simulink model "peak_current_mode_3phase_4quadrant"  (R2021b)
settings: Solver=VariableStepAuto  StartTime=0.0  StopTime=100  RelTol=1e-3
libraries: spsUniversalBridgeLib x2, spsCurrentMeasurementLib x1, spsDCMachineLib x1, spsDCVoltageSourceLib x1, spsThreePhaseVIMeasurementLib x1, spsThreePhaseSourceLib x1, spspowerguiLib x1
settings Model: Creator=Göktuğ  LastModifiedBy=Göktuğ

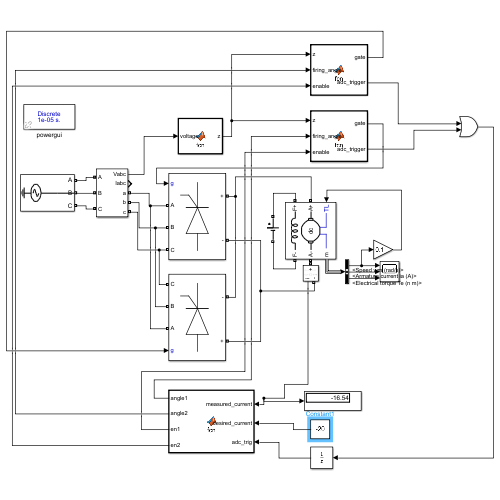
[thumbnail: Simulink's stored preview of the top-level diagram]
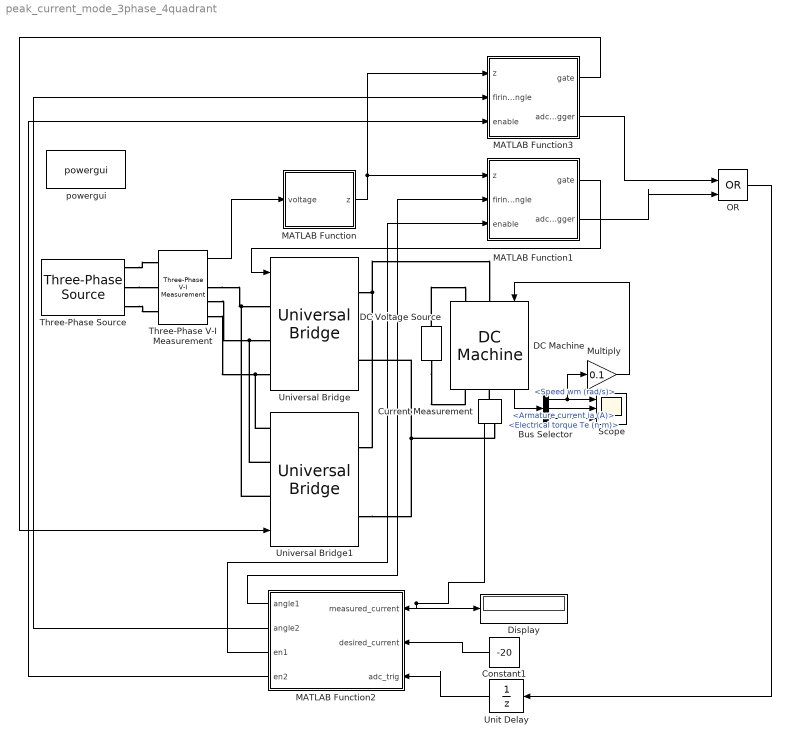
== system peak_current_mode_3phase_4quadrant ==
  Bus Selector : BusSelector  OutputSignals=Speed wm (rad/s),Armature current ia (A),Electrical torque Te (n m)
  Constant1 : Constant  Value=-20
  Current Measurement : spsCurrentMeasurementLib/Current Measurement  PhasorSimulation=off  OutputType=Complex  PSBequivalent=0
  DC Machine : spsDCMachineLib/DC Machine  PresetModel=No  MechanicalLoad=Torque TL  FieldType=Wound  ShowDetailedParameters=on  MeasurementBus=off  RLa="[ 0.8  12.5e-3]"  RLf="[ 240  120]"  Laf=1.8  MachineConstant=Torque constant (N.m/A)  Ke=1.8  Kt=1.8  J=1  Bm=0  Tf=0  w0=0  Ifinit=0.125  TsPowergui=0  TsBlock=-1
  DC Voltage Source : spsDCVoltageSourceLib/DC Voltage Source  Amplitude=150  Measurements=None
  Display : Display
  MATLAB Function : MATLAB Function  TreatAsAtomicUnit=on
  MATLAB Function1 : MATLAB Function  TreatAsAtomicUnit=on
  MATLAB Function2 : MATLAB Function  TreatAsAtomicUnit=on
  MATLAB Function3 : MATLAB Function  TreatAsAtomicUnit=on
  Multiply : Gain  Gain=0.1
  OR : Logic  Operator=OR  IconShape=distinctive  AllPortsSameDT=off  OutDataTypeStr=boolean
  Scope : Scope  NumInputPorts=3
  Three-Phase V-I Measurement : spsThreePhaseVIMeasurementLib/Three-Phase V-I Measurement  VoltageMeasurement=phase-to-ground  SetLabelV=off  LabelV=Vabc  Vpu=off  VpuLL=off  CurrentMeasurement=yes  SetLabelI=off  LabelI=Iabc  Ipu=off  Pbase=100e6  Vbase=500e3  OutputType=Complex  PhasorSimulation=off  PSBequivalent=0
  Three-Phase Source : spsThreePhaseSourceLib/Three-Phase Source  InternalConnection=Yg  VoltagePhases=off  Voltage=180  PhaseAngle=0  Voltage_phases=[25e3 25e3 25e3]/sqrt(3)  PhaseAngles_phases=[0 -120 +120]  Frequency=50  NonIdealSource=on  SpecifyImpedance=off  Resistance=0  Inductance=0  ShortCircuitLevel=100e6  BaseVoltage=0  XRratio=7  BusType=swing  Pref=10e3  Qref=0  Prefabc=[10e3, 10e3, 10e3]  Qrefabc=[0, 0, 0]  Qmin=-inf  Qmax=inf
  Unit Delay : UnitDelay  SampleTime=-1  HasFrameUpgradeWarning=on
  Universal Bridge : spsUniversalBridgeLib/Universal Bridge  Arms=3  SnubberResistance=1e5  SnubberCapacitance=inf  Device=Thyristors  Ron=1e-3  Lon=0  ForwardVoltages="[  0  0  ]"  ForwardVoltage=0  GTOparameters=[ 10e-6 , 20e-6 ]  IGBTparameters=[ 1e-6 , 2e-6 ]  Measurements=None  Measurements_2=None  converterType=Rectifier
  Universal Bridge1 : spsUniversalBridgeLib/Universal Bridge  Arms=3  SnubberResistance=1e5  SnubberCapacitance=inf  Device=Thyristors  Ron=1e-3  Lon=0  ForwardVoltages="[  0  0  ]"  ForwardVoltage=0  GTOparameters=[ 10e-6 , 20e-6 ]  IGBTparameters=[ 1e-6 , 2e-6 ]  Measurements=None  Measurements_2=None  converterType=Rectifier
  powergui : spspowerguiLib/powergui  Priority=1  SimulationMode=Discrete  SampleTime=10e-6  frequency=60  Iterations=50  frequencyindice=0  Pbase=100e6  ErrMax=1e-4  UnitsV=kV  UnitsW=MW  buscounter=0  FunctionMessages=off  echomessages=off  EnableUseOfTLC=off  CurrentSourceSwitches=off  DisableSnubberDevices=off  DisableRonSwitches=off  DisableVfSwitches=off  DisplayEquations=off  AutomaticDiscreteSolvers=off  SolverType=Tustin/Backward Euler (TBE)  Interpol=off  ExternalGateDelay=off  methode=off  Ts=100  x0status=blocks  SPID=on  SwTol=0  HookPort=off  NonlinearTolerance=1e-4  nMaxIteration=100  ContinueOnMaxIteration=off  RestoreLinks=warning  ResistiveCurrentMeasurement=off  Frange=[0:2:500]  Ylog=off  Xlog=on  ShowGrid=off  save=off  variable=ZData  structure=0  ZoomFFT=off  StartTime=0.0  cycles=1  DisplayStyle=1  fundamental=60  FreqAxis=off  MaxFrequency=1000  frequencyindicesteady=1  RmsSteady=1  display=off
  wires:
  MATLAB Function/1(z) -> MATLAB Function3/1(z), MATLAB Function1/1(z)
  MATLAB Function1/1(gate) -> Universal Bridge/1
  Three-Phase V-I Measurement/1 -> MATLAB Function/1(voltage)
  Current Measurement/1 -> Display/1, MATLAB Function2/1(measured_current)
  Constant1/1 -> MATLAB Function2/2(desired_current)
  MATLAB Function2/1(angle1) -> MATLAB Function1/2(firing_angle)
  DC Machine/1 -> Bus Selector/1
  Bus Selector/1 -> Scope/1, Multiply/1  "<Speed wm (rad/s)>"
  Bus Selector/2 -> Scope/2  "<Armature current ia (A)>"
  Bus Selector/3 -> Scope/3  "<Electrical torque Te (n m)>"
  Multiply/1 -> DC Machine/1
  Unit Delay/1 -> MATLAB Function2/3(adc_trig)
  MATLAB Function1/2(adc_trigger) -> OR/2
  MATLAB Function3/2(adc_trigger) -> OR/1
  MATLAB Function3/1(gate) -> Universal Bridge1/1
  OR/1 -> Unit Delay/1
  MATLAB Function2/2(angle2) -> MATLAB Function3/2(firing_angle)
  MATLAB Function2/3(en1) -> MATLAB Function1/3(enable)
  MATLAB Function2/4(en2) -> MATLAB Function3/3(enable)
  connections:
  Three-Phase Source/RConn1 -- Three-Phase V-I Measurement/LConn1
  Three-Phase Source/RConn2 -- Three-Phase V-I Measurement/LConn2
  Three-Phase Source/RConn3 -- Three-Phase V-I Measurement/LConn3
  Three-Phase V-I Measurement/RConn1 -- Universal Bridge1/LConn1 -- Universal Bridge/LConn1
  Three-Phase V-I Measurement/RConn2 -- Universal Bridge1/LConn2 -- Universal Bridge/LConn2
  Three-Phase V-I Measurement/RConn3 -- Universal Bridge1/LConn3 -- Universal Bridge/LConn3
  DC Voltage Source/RConn1 -- DC Machine/LConn2
  DC Voltage Source/LConn1 -- DC Machine/RConn2
  Universal Bridge/RConn1 -- Universal Bridge1/RConn2 -- DC Machine/LConn1
  Current Measurement/LConn1 -- DC Machine/RConn1
  Current Measurement/RConn1 -- Universal Bridge1/RConn1 -- Universal Bridge/RConn2

== matlab function peak_current_mode_3phase_4quadrant/MATLAB Function1 ==
  data: z input; gate output size=[1 6]; firing_angle input; adc_trigger output; enable input
function [gate, adc_trigger]= fcn(z, firing_angle, enable)

persistent angle_pA;

persistent step;

if isempty(step)
    step = 6;
end

if isempty(angle_pA)
    angle_pA = 0;
end

d2r=pi/180;
r2d=180/pi;


if z==1 %sync first phase
    angle_pA = 0;
else
    angle_pA = angle_pA + 0.18;
end

%bridge config is 1 3 5
%                 4 6 2
if (enable == 1)
        if(r2d*angdiff((firing_angle+30)*d2r,angle_pA*d2r)>=0 && r2d*angdiff((firing_angle+90)*d2r,angle_pA*d2r)<0)%step1
            step = 1;
            gate_sig = [1 0 0 0 0 0];
        elseif(r2d*angdiff((firing_angle+90)*d2r,angle_pA*d2r)>=0 && r2d*angdiff((firing_angle+150)*d2r,angle_pA*d2r)<0)%step2
            step = 2;
            gate_sig = [0 1 0 0 0 0];
            elseif(r2d*angdiff((firing_angle+150)*d2r,angle_pA*d2r)>=0 && r2d*angdiff((firing_angle+210)*d2r,angle_pA*d2r)<0)%step3
            step = 3;
            gate_sig = [0 0 1 0 0 0];
        elseif(r2d*angdiff((firing_angle+210)*d2r,angle_pA*d2r)>=0 && r2d*angdiff((firing_angle+270)*d2r,angle_pA*d2r)<0)%step4
            step = 4;
            gate_sig = [0 0 0 1 0 0];
        elseif(r2d*angdiff((firing_angle+270)*d2r,angle_pA*d2r)>=0 && r2d*angdiff((firing_angle+330)*d2r,angle_pA*d2r)<0)%step5
            step = 5;
            gate_sig = [0 0 0 0 1 0];
        elseif(r2d*angdiff((firing_angle+330)*d2r,angle_pA*d2r)>=0 && r2d*angdiff((firing_angle+30)*d2r,angle_pA*d2r)<0)%step6
            step = 6;
            gate_sig = [0 0 0 0 0 1];
        else
            gate_sig = [0 0 0 0 0 0];
        end
        if(r2d*angdiff((firing_angle+59.5)*d2r,angle_pA*d2r)>=0 && r2d*angdiff((firing_angle+60.5)*d2r,angle_pA*d2r)<0)%step1
            adc = 1;
        elseif(r2d*angdiff((firing_angle+119.5)*d2r,angle_pA*d2r)>=0 && r2d*angdiff((firing_angle+120.5)*d2r,angle_pA*d2r)<0)%step2
            adc = 1;
        elseif(r2d*angdiff((firing_angle+179.5)*d2r,angle_pA*d2r)>=0 && r2d*angdiff((firing_angle+180.5)*d2r,angle_pA*d2r)<0)%step3
            adc = 1;
        elseif(r2d*angdiff((firing_angle+239.5)*d2r,angle_pA*d2r)>=0 && r2d*angdiff((firing_angle+240.5)*d2r,angle_pA*d2r)<0)%step4
            adc = 1;
        elseif(r2d*angdiff((firing_angle+300.5)*d2r,angle_pA*d2r)>=0 && r2d*angdiff((firing_angle+301.5)*d2r,angle_pA*d2r)<0)%step5
            adc = 1;
        elseif(r2d*angdiff((firing_angle+359.5)*d2r,angle_pA*d2r)>=0 && r2d*angdiff((firing_angle+0.5)*d2r,angle_pA*d2r)<0)%step6
            adc = 1;
        else
            adc = 0;
        end
else
    gate_sig = [0 0 0 0 0 0];
    adc = 0;
end
gate = gate_sig;
adc_trigger = adc;
end

== matlab function peak_current_mode_3phase_4quadrant/MATLAB Function ==
  data: voltage input; z output
function z   = fcn( voltage)
    
    persistent past_voltage;
    
    if isempty(past_voltage)
        past_voltage = 0;
    end

    if(past_voltage < 0 && voltage(1)>=0)
        z=1;
    else
        z=0;
    end
    past_voltage = voltage(1);
end

== matlab function peak_current_mode_3phase_4quadrant/MATLAB Function2 ==
  data: measured_current input; desired_current input; angle1 output; angle2 output; en1 output; en2 output; adc_trig input
function [angle1, angle2, en1, en2]= fcn(measured_current,desired_current, adc_trig)
persistent firing_angle1;
persistent firing_angle2;

if(isempty(firing_angle1))
    firing_angle1 = 120;
end
if(isempty(firing_angle2))
    firing_angle2 = 120;
end

if desired_current>0%angle1 enable1
    if(adc_trig == 1)
        if(desired_current>measured_current)
            firing_angle1 = firing_angle1 - 0.05;
        elseif(measured_current>desired_current)
            firing_angle1 = firing_angle1 + 0.05;
        end
        if(firing_angle1<0)
            firing_angle1 = 0;
        elseif(firing_angle1>120)
            firing_angle1=120;
        end
    
    end
        firing_angle2 = 120;
        angle1 = firing_angle1;
        en1=1;
        angle2=120;
        en2=0;
elseif desired_current<0%angle2 enable2
      if(adc_trig == 1)
        if(desired_current<measured_current)
            firing_angle2 = firing_angle2 - 0.05;
        elseif(measured_current<desired_current)
            firing_angle2 = firing_angle2 + 0.05;
        end
        if(firing_angle2<0)
            firing_angle2 = 0;
        elseif(firing_angle2>120)
            firing_angle2=120;
        end
    
      end
        firing_angle1 = 120;
        angle1 = 120;
        en1=0;
        angle2 = firing_angle2;
        en2=1;
else
en1=0;
en2=0;
angle1=0;
angle2=0;
end

end

== matlab function peak_current_mode_3phase_4quadrant/MATLAB Function3 ==
  data: z input; gate output size=[1 6]; firing_angle input; adc_trigger output; enable input
function [gate, adc_trigger]= fcn(z, firing_angle, enable)

persistent angle_pA;

persistent step;

if isempty(step)
    step = 6;
end

if isempty(angle_pA)
    angle_pA = 0;
end

d2r=pi/180;
r2d=180/pi;


if z==1 %sync first phase
    angle_pA = 0;
else
    angle_pA = angle_pA + 0.18;
end

%bridge config is 1 3 5
%                 4 6 2
if (enable == 1)
        if(r2d*angdiff((firing_angle+30)*d2r,angle_pA*d2r)>=0 && r2d*angdiff((firing_angle+90)*d2r,angle_pA*d2r)<0)%step1
            step = 1;
            gate_sig = [1 0 0 0 0 0];
        elseif(r2d*angdiff((firing_angle+90)*d2r,angle_pA*d2r)>=0 && r2d*angdiff((firing_angle+150)*d2r,angle_pA*d2r)<0)%step2
            step = 2;
            gate_sig = [0 1 0 0 0 0];
            elseif(r2d*angdiff((firing_angle+150)*d2r,angle_pA*d2r)>=0 && r2d*angdiff((firing_angle+210)*d2r,angle_pA*d2r)<0)%step3
            step = 3;
            gate_sig = [0 0 1 0 0 0];
        elseif(r2d*angdiff((firing_angle+210)*d2r,angle_pA*d2r)>=0 && r2d*angdiff((firing_angle+270)*d2r,angle_pA*d2r)<0)%step4
            step = 4;
            gate_sig = [0 0 0 1 0 0];
        elseif(r2d*angdiff((firing_angle+270)*d2r,angle_pA*d2r)>=0 && r2d*angdiff((firing_angle+330)*d2r,angle_pA*d2r)<0)%step5
            step = 5;
            gate_sig = [0 0 0 0 1 0];
        elseif(r2d*angdiff((firing_angle+330)*d2r,angle_pA*d2r)>=0 && r2d*angdiff((firing_angle+30)*d2r,angle_pA*d2r)<0)%step6
            step = 6;
            gate_sig = [0 0 0 0 0 1];
        else
            gate_sig = [0 0 0 0 0 0];
        end
        if(r2d*angdiff((firing_angle+59.5)*d2r,angle_pA*d2r)>=0 && r2d*angdiff((firing_angle+60.5)*d2r,angle_pA*d2r)<0)%step1
            adc = 1;
        elseif(r2d*angdiff((firing_angle+119.5)*d2r,angle_pA*d2r)>=0 && r2d*angdiff((firing_angle+120.5)*d2r,angle_pA*d2r)<0)%step2
            adc = 1;
        elseif(r2d*angdiff((firing_angle+179.5)*d2r,angle_pA*d2r)>=0 && r2d*angdiff((firing_angle+180.5)*d2r,angle_pA*d2r)<0)%step3
            adc = 1;
        elseif(r2d*angdiff((firing_angle+239.5)*d2r,angle_pA*d2r)>=0 && r2d*angdiff((firing_angle+240.5)*d2r,angle_pA*d2r)<0)%step4
            adc = 1;
        elseif(r2d*angdiff((firing_angle+300.5)*d2r,angle_pA*d2r)>=0 && r2d*angdiff((firing_angle+301.5)*d2r,angle_pA*d2r)<0)%step5
            adc = 1;
        elseif(r2d*angdiff((firing_angle+359.5)*d2r,angle_pA*d2r)>=0 && r2d*angdiff((firing_angle+0.5)*d2r,angle_pA*d2r)<0)%step6
            adc = 1;
        else
            adc = 0;
        end
else
    gate_sig = [0 0 0 0 0 0];
    adc = 0;
end
gate = gate_sig;
adc_trigger = adc;
end
